simulink model "lab2"  (R2021b)
settings: Solver=VariableStepAuto  StartTime=0.0  StopTime=10.0  RelTol=1e-3
settings Model: Creator=arek  LastModifiedBy=arek

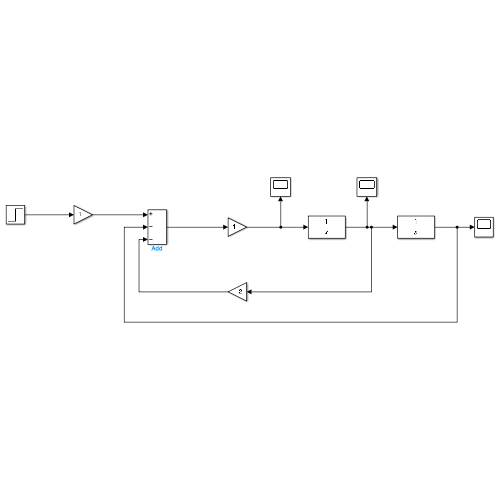
[thumbnail: Simulink's stored preview of the top-level diagram]
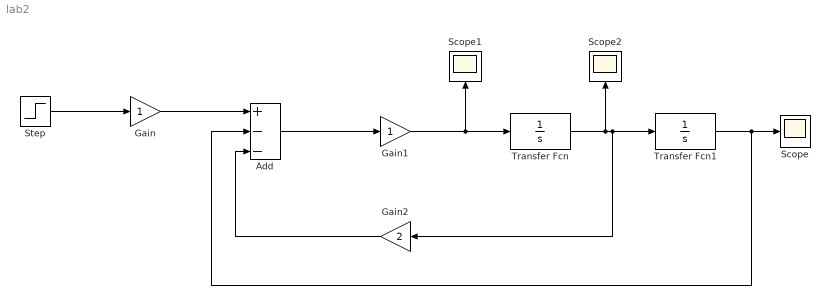
== system lab2 ==
  Add : Sum  Inputs=+--
  Gain : Gain
  Gain1 : Gain
  Gain2 : Gain  Gain=2
  Scope : Scope
  Scope1 : Scope
  Scope2 : Scope
  Step : Step  SampleTime=0
  Transfer Fcn : TransferFcn  Denominator=[1 0]
  Transfer Fcn1 : TransferFcn  Denominator=[1 0]
  wires:
  Step/1 -> Gain/1
  Gain/1 -> Add/1
  Add/1 -> Gain1/1
  Gain1/1 -> Scope1/1, Transfer Fcn/1
  Transfer Fcn/1 -> Scope2/1, Gain2/1, Transfer Fcn1/1
  Gain2/1 -> Add/3
  Transfer Fcn1/1 -> Add/2, Scope/1
